simulink model "DCM_N_to_B"  (R2021b)
settings: Solver=VariableStepAuto  StartTime=0.0  StopTime=SimTime  MaxStep=1e-2  RelTol=1e-13
values from neighbouring files (symbols this model uses):
  A0 = [sqrt(2) sqrt(2) 0 ... (first row only)    [Lab_4.m]    (also in Lab_6.m = eye(3))
libraries: robotcorelib x1, sharedutil x1
settings Model: Creator=adity  LastModifiedBy=adity
settings SolverCC: AlgebraicLoopSolver=TrustRegion
settings DebuggingCC: SFMachineParentedDataDiag=warning

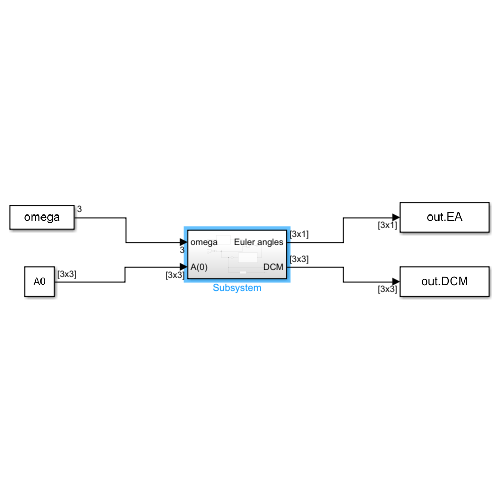
[thumbnail: Simulink's stored preview of the top-level diagram]
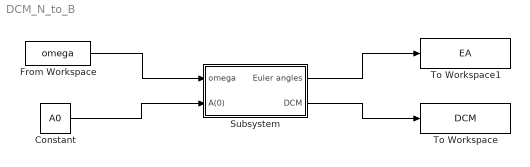
== system DCM_N_to_B ==
  Constant : Constant  Value=A0
  From Workspace : FromWorkspace  VariableName=omega
  Subsystem : Subsystem
  To Workspace : ToWorkspace  VariableName=DCM  SaveFormat=Timeseries  SampleTime=-1
  To Workspace1 : ToWorkspace  VariableName=EA  SaveFormat=Timeseries  SampleTime=-1
  wires:
  From Workspace/1 -> Subsystem/1(omega)
  Constant/1 -> Subsystem/2(A(0))
  Subsystem/2(DCM) -> To Workspace/1
  Subsystem/1(Euler angles) -> To Workspace1/1

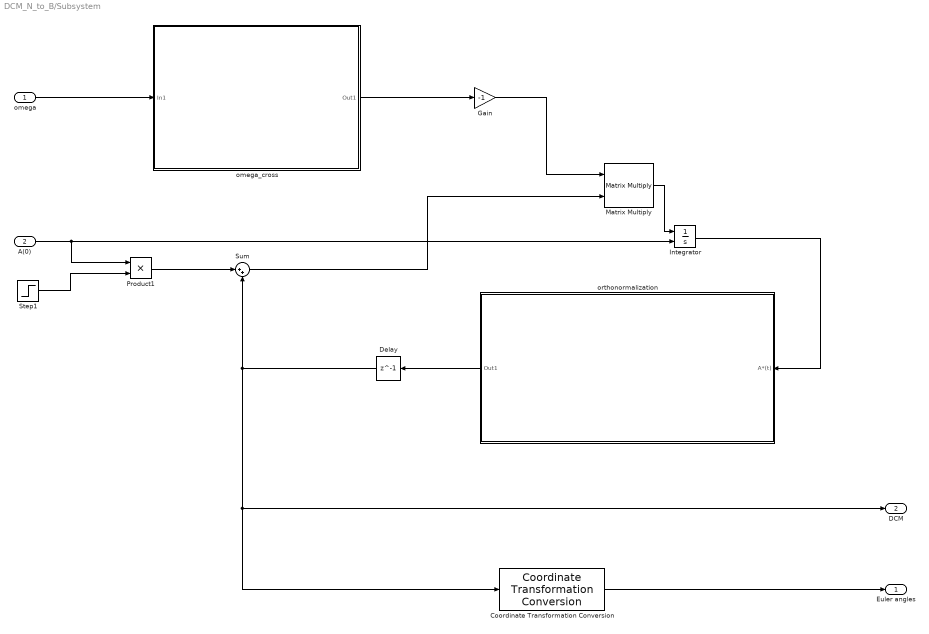
== system DCM_N_to_B/Subsystem ==
  omega : Inport
  A(0) : Inport  Port=2
  Coordinate Transformation Conversion : robotcorelib/Coordinate Transformation Conversion  InputRepresentation=Rotation Matrix  InputEulerSequence=ZYX  ShowTrVecInputPort=on  OutputRepresentation=Euler Angles  OutputEulerSequence=ZYZ  ShowTrVecOutputPort=on  SimulateUsing=Interpreted execution
      settings: SourceProductBaseCode=NV,RO,RR,UV
  Delay : Delay  DelayLength=1
  Gain : Gain  Gain=-1
  Integrator : Integrator  InitialConditionSource=external  InitialCondition=A0
  Matrix Multiply : Product  Multiplication=Matrix(*)
  Product1 : Product
  Step1 : Step  Time=0.01  Before=1  After=0  SampleTime=0
  Sum : Sum  Inputs=|++
  "omega_cross " : Subsystem
  orthonormalization : Subsystem
  Euler angles : Outport
  DCM : Outport  Port=2
  wires:
  Matrix Multiply/1 -> Integrator/1
  A(0)/1 -> Integrator/2, Product1/1
  Gain/1 -> Matrix Multiply/1
  "omega_cross "/1(Out1) -> Gain/1
  orthonormalization/1(Out1) -> Delay/1
  Step1/1 -> Product1/2
  Integrator/1 -> orthonormalization/1(A*(t))
  omega/1 -> "omega_cross "/1(In1)
  Coordinate Transformation Conversion/1 -> Euler angles/1
  Product1/1 -> Sum/1
  Delay/1 -> Sum/2, DCM/1, Coordinate Transformation Conversion/1
  Sum/1 -> Matrix Multiply/2

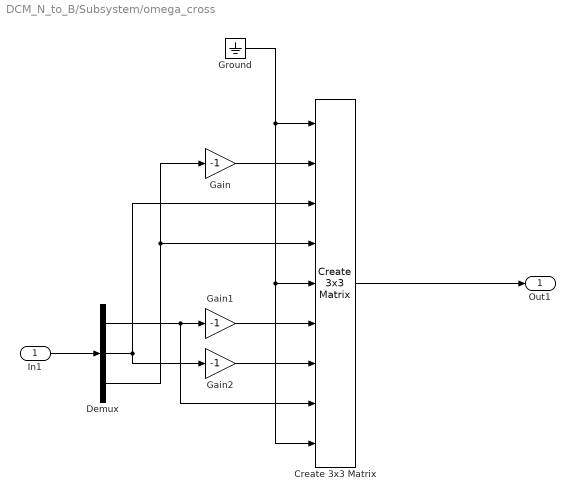
== system DCM_N_to_B/Subsystem/omega_cross  ==
  In1 : Inport
  Create 3x3 Matrix : sharedutil/Create 3x3 Matrix  aMode=aMode
      settings: SourceProductBaseCode=AE,PW,DR,MT,UV,VE
  Demux : Demux  Outputs=3
  Gain : Gain  Gain=-1
  Gain1 : Gain  Gain=-1
  Gain2 : Gain  Gain=-1
  Ground : Ground
  Out1 : Outport
  wires:
  In1/1 -> Demux/1
  Ground/1 -> Create 3x3 Matrix/5, Create 3x3 Matrix/9, Create 3x3 Matrix/1
  Gain/1 -> Create 3x3 Matrix/2
  Gain1/1 -> Create 3x3 Matrix/6
  Gain2/1 -> Create 3x3 Matrix/7
  Demux/3 -> Gain/1, Create 3x3 Matrix/4
  Demux/2 -> Gain2/1, Create 3x3 Matrix/3
  Demux/1 -> Gain1/1, Create 3x3 Matrix/8
  Create 3x3 Matrix/1 -> Out1/1

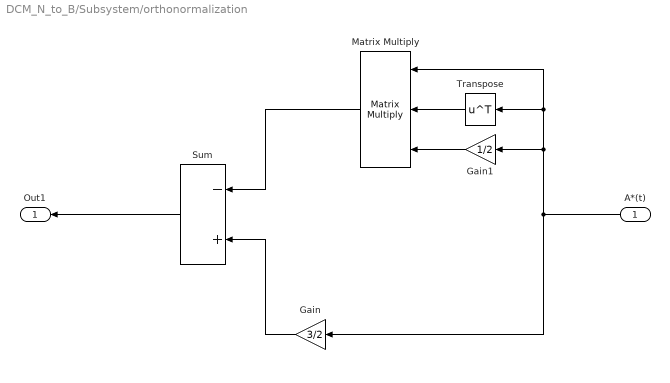
== system DCM_N_to_B/Subsystem/orthonormalization ==
  A*(t) : Inport
  Gain : Gain  Gain=3/2
  Gain1 : Gain  Gain=1/2
  Matrix Multiply : Product  Inputs=3  Multiplication=Matrix(*)
  Sum : Sum  Inputs=-+
  Transpose : Math  Operator=transpose  SaturateOnIntegerOverflow=on
  Out1 : Outport
  wires:
  A*(t)/1 -> Matrix Multiply/1, Transpose/1, Gain1/1, Gain/1
  Sum/1 -> Out1/1
  Gain/1 -> Sum/2
  Transpose/1 -> Matrix Multiply/2
  Gain1/1 -> Matrix Multiply/3
  Matrix Multiply/1 -> Sum/1
